simulink model "testsimulinkmodel"  (R2019a)
settings: Solver=VariableStepAuto  StartTime=0.0  StopTime=10.0  RelTol=1e-3
settings Model: Creator=paalthorseth  LastModifiedBy=paalthorseth

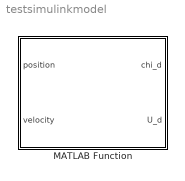
== system testsimulinkmodel ==
  MATLAB Function : MATLAB Function  TreatAsAtomicUnit=on

== matlab function testsimulinkmodel/MATLAB Function ==
  data: position input; chi_d output; velocity input; U_d output
function [chi_d, U_d]= Lookahead_LOS_Guidance(position,velocity)

persistent init_flag n K_p;

if isempty(init_flag)
    % Load waypoints
    load('../Matlab/WP.mat');
    
    % Define waypoint n
    n   = 1;
    
    % Controller parameters
    Delta   = 500;
    K_p     = 1/Delta;
    
    init_flag = 1;
end


% Define variables
x       = position(1);     % position x in NED
y       = position(2);     % position y in NED

u       = velocity(1);     % velocity u in BODY
v       = velocity(2);     % velocity v in BODY

% Current waypoint
x_wp_c  = WP(n,1);
y_wp_c  = WP(n,2);

% Next waypoint
x_wp_n  = WP(n+1,1);
y_wp_n  = WP(n+1,2);

% Path-tangential angle
alpha   = atan2(y_wp_n - y_wp_c, x_wp_n - x_wp_c);

% Cross-track error
e       = - (x - x_wp_c)*sin(alpha) + (y - y_wp_c)*cos(alpha);

% Define course reference 
chi_p   = alpha;
chi_r   = arctan(-K_p*e);
chi_d   = chi_p + chi_r;

% Radius for circle of acceptance
R       = 2*304.8; 

% Check circle of acceptance
if ((x_wp_n - x)^2 + (y_wp_n - y)^2) <= R
    n   = n + 1;        % Update waypoint
end


% Set desired speed
U_d     = 3;            % [m/s]
